simulink model "HFI_UB_counter_latch"  (R2024a)
settings: Solver=FixedStepAuto  StartTime=0.0  StopTime=10  FixedStep=1e-6  RelTol=1e-3
values from neighbouring files (symbols this model uses):
  flux = 0.005753    [HFI_AVi.sldd]
  Ld = 0.00025    [HFI_AVi.sldd]
  Lq = 0.00056    [HFI_AVi.sldd]
  R = 0.6    [HFI_AVi.sldd]
undefined symbols (not defined in the file or in its folder): DiscIntNeverNeededParam, PI
libraries: simulink x3, slpidlib x3, powerlib_extras x2, spsDCVoltageSourceLib x1, spsGroundLib x1, spsPermanentMagnetSynchronousMachineLib x1, spsUniversalBridgeLib x1, sps_lib x1
(part 2 of 2)

== system HFI_UB_counter_latch/FOC_Model/currloop/求定子电流矢量角/Id ~=0/id1<=0 ==
  In1 : Inport
  Action Port : ActionPort  ActionPortLabel=if(u1 <= 0)
  Out1 : Outport
  wires:
  In1/1 -> Out1/1

== system HFI_UB_counter_latch/FOC_Model/currloop/求定子电流矢量角/Id ~=0/id1>0 ==
  In1 : Inport
  Action Port : ActionPort  ActionPortLabel=else
  Out1 : Outport
  wires:
  In1/1 -> Out1/1

== system HFI_UB_counter_latch/FOC_Model/currloop/求定子电流矢量角/Id ~=0/id<=0 ==
  In1 : Inport
  Action Port : ActionPort  ActionPortLabel=if(u1 <= 0)
  Out1 : Outport
  wires:
  In1/1 -> Out1/1

== system HFI_UB_counter_latch/FOC_Model/currloop/求定子电流矢量角/Id ~=0/id>0 ==
  In1 : Inport
  Action Port : ActionPort  ActionPortLabel=else
  Out1 : Outport
  wires:
  In1/1 -> Out1/1

== matlab function HFI_UB_counter_latch/FOC_Model/currloop/polo/Subsystem4/CounterLatch150ms ==
  data: u input; y output
function y = fcn(u)
%#codegen
% Capture u once at 150 ms (Ts = 100 us) and hold it.
persistent sample_count latched_value
if isempty(sample_count)
    sample_count = uint16(0);
    latched_value = single(0);
end
if sample_count == uint16(1500)
    latched_value = single(u);
end
if sample_count < uint16(1501)
    sample_count = sample_count + uint16(1);
end
y = latched_value;
end

== matlab function HFI_UB_counter_latch/FOC_Model/currloop/SVPWM MATLAB Function ==
  data: Valpha input single size=1; Tcmp1 output single size=1; Vbeta input single size=1; Tcmp2 output single size=1; Tcmp3 output single size=1; Udc input single size=1; Tpwm input single size=1; sector output single size=1
function [Tcmp1,Tcmp2,Tcmp3,sector] = fcn(Valpha,Vbeta,Udc,Tpwm)
%#codegen

sector = single(0);
Tcmp1 = single(0);
Tcmp2 = single(0);
Tcmp3 = single(0);

%========Parameters statement================

    Vref1 = Vbeta;							                   
    Vref2 = (sqrt(3)*Valpha - Vbeta)/2; 				    
    Vref3 = (-sqrt(3)*Valpha - Vbeta)/2;					
   
 %========Sector calculation=================

  if (Vref1>0)
	   sector = single(1);
  end
  if (Vref2>0)
	   sector = sector+single(2);
  end
  if (Vref3>0)
       sector = sector+single(4);
  end

%======== X Y Z calculation===================

X = sqrt(3)*Vbeta*Tpwm/Udc;
Y = Tpwm/Udc*(3/2*Valpha+sqrt(3)/2*Vbeta);
Z = Tpwm/Udc*(-3/2*Valpha+sqrt(3)/2*Vbeta);	         

%==========Duty ratio calculation================
switch (sector)   
    case 1
        T1 = Z; T2 = Y; 
	case 2
        T1 = Y; T2 = -X; 
	case 3
        T1 = -Z; T2 = X; 
	case 4
        T1 = -X; T2 = Z;
	case 5
        T1 = X; T2 = -Y;
    otherwise
        T1 = -Y; T2 = -Z;
end

if T1+T2 > Tpwm
    T1 = T1/(T1+T2);
    T2 = T2/(T1+T2);
else
    T1 = T1;
    T2 = T2;
end
ta = (Tpwm-(T1+T2))/4.0;
tb = ta+T1/2;
tc = tb+T2/2;

%==========Duty ratio calculation================
switch (sector)
    case 1 
        Tcmp1=tb;
        Tcmp2=ta;
        Tcmp3=tc; 
        
    case 2 
        Tcmp1=ta;
        Tcmp2=tc;
        Tcmp3=tb; 
       
    case 3 
        Tcmp1=ta;
        Tcmp2=tb;
        Tcmp3=tc; 
        
    case 4 
        Tcmp1=tc;
        Tcmp2=tb;
        Tcmp3=ta;
        
    case 5 
        Tcmp1=tc;
        Tcmp2=ta;
        Tcmp3=tb;
        
   case 6
       Tcmp1=tb;
       Tcmp2=tc;
       Tcmp3=ta;
end
end

== matlab function HFI_UB_counter_latch/FOC_Model/currloop/MATLAB Function ==
  data: model_n input single size=1; hf_n input single size=1; n output single size=1; model_thetae input; hfi_thetae input; t input; thetae output; flag output; hfi_ready output; mode_out output
function [n, thetae, flag, hfi_ready, mode_out] = fcn( ...
    model_n, hf_n, model_thetae, hfi_thetae, t)
%#codegen

%% ================= 参数 =================
TS = single(1e-4);             % 100 us，10 kHz

HFI_BLEND_START = single(300); % 开始HFI-SMO融合
SMO_ENTER       = single(700); % 700 r/min以上才进入纯SMO
SMO_EXIT        = single(550); % 550 r/min以下退出纯SMO

ANGLE_MAX = single(pi/6);      % 最大角度差30°
SPEED_MAX = single(150);       % 最大速度差150 r/min

ENTER_CONFIRM = uint16(100);   % 10 ms
EXIT_CONFIRM  = uint16(100);   % 10 ms
VALID_CONFIRM = uint16(50);    % 5 ms
WAKE_SAMPLES  = uint16(200);   % 20 ms

T_BLEND     = single(0.05);    % 50 ms融合时间
LAMBDA_STEP = TS/T_BLEND;

PI     = single(pi);
TWO_PI = single(2*pi);

% mode:
% 0 = 纯HFI
% 1 = HFI向SMO融合
% 2 = 纯SMO
% 3 = HFI预唤醒，输出仍使用SMO
% 4 = SMO向HFI融合

%% ================= 状态变量 =================
persistent mode
persistent lambda_mem
persistent theta_prev
persistent enter_count
persistent exit_count
persistent valid_count
persistent wake_count

if isempty(mode)
    mode = uint8(0);
end

if isempty(lambda_mem)
    lambda_mem = single(0);
end

if isempty(theta_prev)
    theta_prev = single(0);
end

if isempty(enter_count)
    enter_count = uint16(0);
end

if isempty(exit_count)
    exit_count = uint16(0);
end

if isempty(valid_count)
    valid_count = uint16(0);
end

if isempty(wake_count)
    wake_count = uint16(0);
end

%% ============ HFI与SMO一致性检查 ============

% 最短角度差，范围为-pi～pi
dtheta = model_thetae - hfi_thetae;
dtheta = mod(dtheta + PI, TWO_PI) - PI;

angle_valid = abs(dtheta) < ANGLE_MAX;
speed_valid = abs(model_n - hf_n) < SPEED_MAX;

estimate_valid = angle_valid && speed_valid;

%% ================= 默认输出 =================
flag      = single(0);
hfi_ready = single(0);

%% ================= 启动阶段 =================
if t < single(0.3)

    mode       = uint8(0);
    lambda_mem = single(0);

    enter_count = uint16(0);
    exit_count  = uint16(0);
    valid_count = uint16(0);
    wake_count  = uint16(0);

    flag      = single(0);  % 完整HFI注入
    hfi_ready = single(1);

    theta_prev = hfi_thetae;

else

    switch mode

        %% ================ 纯HFI ================
        case 0

            lambda_mem = single(0);
            flag       = single(0);
            hfi_ready  = single(1);

            % 达到融合速度，而且两种观测器一致
            if abs(hf_n) >= HFI_BLEND_START && estimate_valid

                if enter_count < ENTER_CONFIRM
                    enter_count = enter_count + uint16(1);
                end

            else
                enter_count = uint16(0);
            end

            % 连续满足10 ms后进入融合
            if enter_count >= ENTER_CONFIRM

                mode = uint8(1);

                enter_count = uint16(0);
                valid_count = uint16(0);
            end

        %% ============ HFI向SMO融合 =============
        case 1

            hfi_ready = single(1);

            % 根据HFI速度计算目标融合权重
            x = (abs(hf_n) - HFI_BLEND_START)/ ...
                (SMO_ENTER - HFI_BLEND_START);

            x = min(max(x, single(0)), single(1));

            % 余弦平滑权重
            lambda_target = single(0.5) - ...
                single(0.5)*cos(PI*x);

            % 两种估算一致时才允许向目标权重变化
            if estimate_valid

                if lambda_mem < lambda_target

                    lambda_mem = min( ...
                        lambda_mem + LAMBDA_STEP, ...
                        lambda_target);

                elseif lambda_mem > lambda_target

                    lambda_mem = max( ...
                        lambda_mem - LAMBDA_STEP, ...
                        lambda_target);
                end

            else
                % 不一致时退回HFI
                lambda_mem = max( ...
                    lambda_mem - LAMBDA_STEP, ...
                    single(0));
            end

            % 解耦HFI注入幅值和角度融合权重：
            % lambda小于0.5时保持完整HFI注入；
            % lambda从0.5到1时再逐渐关闭HFI。
            if lambda_mem <= single(0.5)

                flag = single(0);

            else

                inject_x = ...
                    (lambda_mem-single(0.5))/single(0.5);

                inject_x = min(max( ...
                    inject_x, single(0)), single(1));

                flag = single(0.5) - ...
                    single(0.5)*cos(PI*inject_x);
            end

            % 满足条件后进入纯SMO
            if lambda_mem >= single(0.999) && ...
               abs(model_n) >= SMO_ENTER && ...
               estimate_valid

                if valid_count < VALID_CONFIRM
                    valid_count = valid_count + uint16(1);
                end

            else
                valid_count = uint16(0);
            end

            if valid_count >= VALID_CONFIRM

                mode       = uint8(2);
                lambda_mem = single(1);

                valid_count = uint16(0);
                exit_count  = uint16(0);

                flag      = single(1);
                hfi_ready = single(0);
            end

            % 速度重新降低时退回纯HFI
            if abs(hf_n) < HFI_BLEND_START && ...
               lambda_mem <= single(0.001)

                mode       = uint8(0);
                lambda_mem = single(0);

                enter_count = uint16(0);
                valid_count = uint16(0);
            end

        %% ================= 纯SMO ================
        case 2

            lambda_mem = single(1);
            flag       = single(1); % HFI关闭
            hfi_ready  = single(0);

            % 低于退出阈值持续10 ms
            if abs(model_n) < SMO_EXIT

                if exit_count < EXIT_CONFIRM
                    exit_count = exit_count + uint16(1);
                end

            else
                exit_count = uint16(0);
            end

            if exit_count >= EXIT_CONFIRM

                mode = uint8(3);

                exit_count  = uint16(0);
                wake_count  = uint16(0);
                valid_count = uint16(0);
                enter_count = uint16(0);
            end

        %% =============== HFI预唤醒 ===============
        case 3

            % 仍完全采用SMO角度
            lambda_mem = single(1);
            hfi_ready  = single(0);

            if wake_count < WAKE_SAMPLES
                wake_count = wake_count + uint16(1);
            end

            wake_x = single(wake_count)/ ...
                single(WAKE_SAMPLES);

            wake_x = min(max( ...
                wake_x, single(0)), single(1));

            wake_weight = single(0.5) - ...
                single(0.5)*cos(PI*wake_x);

            % flag从1降到0，HFI注入逐渐恢复
            flag = single(1)-wake_weight;

            % 如果速度重新升高，取消返回HFI
            if abs(model_n) >= SMO_ENTER

                if enter_count < ENTER_CONFIRM
                    enter_count = enter_count + uint16(1);
                end

            else
                enter_count = uint16(0);
            end

            if enter_count >= ENTER_CONFIRM

                mode       = uint8(2);
                lambda_mem = single(1);

                flag       = single(1);
                hfi_ready  = single(0);

                enter_count = uint16(0);
                wake_count  = uint16(0);
                valid_count = uint16(0);

            elseif wake_count >= WAKE_SAMPLES

                % HFI已经恢复，等待估算结果连续一致
                flag = single(0);

                if estimate_valid

                    if valid_count < VALID_CONFIRM
                        valid_count = valid_count + uint16(1);
                    end

                else
                    valid_count = uint16(0);
                end

                if valid_count >= VALID_CONFIRM

                    mode       = uint8(4);
                    lambda_mem = single(1);
                    hfi_ready  = single(1);

                    valid_count = uint16(0);
                end
            end

        %% ============ SMO向HFI融合 =============
        case 4

            flag      = single(0); % 保持完整HFI注入
            hfi_ready = single(1);

            if estimate_valid

                % 两种估算一致时才向HFI平滑切换
                lambda_mem = max( ...
                    lambda_mem-LAMBDA_STEP, ...
                    single(0));

            else
                % HFI失去可信度时停止切换，
                % 返回预唤醒/一致性确认状态
                mode       = uint8(3);
                lambda_mem = single(1);

                wake_count  = WAKE_SAMPLES;
                valid_count = uint16(0);

                flag      = single(0);
                hfi_ready = single(0);
            end

            if lambda_mem <= single(0.001)

                mode       = uint8(0);
                lambda_mem = single(0);

                enter_count = uint16(0);
                valid_count = uint16(0);
            end

        otherwise

            mode       = uint8(0);
            lambda_mem = single(0);

            enter_count = uint16(0);
            exit_count  = uint16(0);
            valid_count = uint16(0);
            wake_count  = uint16(0);

            flag      = single(0);
            hfi_ready = single(1);
    end
end

%% ================= 速度融合 =================
n = (single(1)-lambda_mem)*hf_n + ...
    lambda_mem*model_n;

%% ================= 角度融合 =================

% dtheta是HFI到SMO的最短角度差
theta_candidate = hfi_thetae + ...
    lambda_mem*dtheta;

%% ============== 保证输出角度连续 ==============

candidate_wrapped = mod(theta_candidate, TWO_PI);
previous_wrapped  = mod(theta_prev, TWO_PI);

theta_step = candidate_wrapped - previous_wrapped;
theta_step = mod(theta_step + PI, TWO_PI) - PI;

theta_continuous = theta_prev + theta_step;
theta_prev       = theta_continuous;

% Park变换继续使用0～2pi范围内的电角度
thetae = mod(theta_continuous, TWO_PI);

%% ================= 调试输出 =================
mode_out = single(mode);

end

== matlab function HFI_UB_counter_latch/FOC_Model/currloop/DirectionLatch ==
  data: hf_n input; direction output; hfi_ready input
function direction = fcn(hf_n, hfi_ready)
%#codegen

persistent dir_mem
persistent positive_count
persistent negative_count

if isempty(dir_mem)
    dir_mem = single(1);
end

if isempty(positive_count)
    positive_count = uint16(0);
end

if isempty(negative_count)
    negative_count = uint16(0);
end

SPEED_THRESHOLD = single(50);
CONFIRM_COUNT = uint16(50); % 5 ms，模块按10 kHz执行

if hfi_ready > single(0.5)

    if hf_n > SPEED_THRESHOLD

        negative_count = uint16(0);

        if positive_count < CONFIRM_COUNT
            positive_count = positive_count + uint16(1);
        end

        if positive_count >= CONFIRM_COUNT
            dir_mem = single(1);
        end

    elseif hf_n < -SPEED_THRESHOLD

        positive_count = uint16(0);

        if negative_count < CONFIRM_COUNT
            negative_count = negative_count + uint16(1);
        end

        if negative_count >= CONFIRM_COUNT
            dir_mem = single(-1);
        end

    else
        positive_count = uint16(0);
        negative_count = uint16(0);
    end

else
    positive_count = uint16(0);
    negative_count = uint16(0);
end

direction = dir_mem;

end

== matlab function HFI_UB_counter_latch/MATLAB Function ==
  data: carrier input; g output; Tcm1 input; Tcm2 input; Tcm3 input; db input
function g = fcn(carrier, Tcm1, Tcm2, Tcm3, db)
%#codegen
% 三相中心对齐PWM死区生成
%
% 输入：
%   carrier  三角载波，范围为0～Tpwm/2，单位：s
%   Tcm1     A相比较值，单位：s
%   Tcm2     B相比较值，单位：s
%   Tcm3     C相比较值，单位：s
%   db       实际死区时间，单位：s
%
% 输出：
%   g(1) = A相上管
%   g(2) = A相下管
%   g(3) = B相上管
%   g(4) = B相下管
%   g(5) = C相上管
%   g(6) = C相下管
%
% 原理：
%   carrier >= Tcm + db/2：上管导通
%   carrier <= Tcm - db/2：下管导通
%   中间宽度为db的区域：上下管全部关闭
%
% 因此输入db=1e-6时，实际死区为1 μs。

%% 初始化输出

g = zeros(6,1);

% 防止输入负的死区时间
if db < 0
    db = 0;
end

% 比较值两侧各移动半个死区时间
half_db = db / 2;

%% A相桥臂

if carrier >= (Tcm1 + half_db)

    % A相上管导通，下管关闭
    g(1) = 1;
    g(2) = 0;

elseif carrier <= (Tcm1 - half_db)

    % A相上管关闭，下管导通
    g(1) = 0;
    g(2) = 1;

else

    % 死区期间上下管全部关闭
    g(1) = 0;
    g(2) = 0;

end

%% B相桥臂

if carrier >= (Tcm2 + half_db)

    % B相上管导通，下管关闭
    g(3) = 1;
    g(4) = 0;

elseif carrier <= (Tcm2 - half_db)

    % B相上管关闭，下管导通
    g(3) = 0;
    g(4) = 1;

else

    % 死区期间上下管全部关闭
    g(3) = 0;
    g(4) = 0;

end

%% C相桥臂

if carrier >= (Tcm3 + half_db)

    % C相上管导通，下管关闭
    g(5) = 1;
    g(6) = 0;

elseif carrier <= (Tcm3 - half_db)

    % C相上管关闭，下管导通
    g(5) = 0;
    g(6) = 1;

else

    % 死区期间上下管全部关闭
    g(5) = 0;
    g(6) = 0;

end

end

== matlab function HFI_UB_counter_latch/MATLAB Function1 ==
  data: MtrPos input; actual_deg output; thetae input; est_deg output; error_deg output
function [actual_deg, est_deg, error_deg] = fcn(MtrPos, thetae)
%#codegen

Pn = single(4);
PI = single(pi);
TWO_PI = single(2*pi);

% 电机实际机械角度 → 实际电角度
theta_actual_e = mod(Pn*MtrPos, TWO_PI);

% 观测器电角度
theta_est_e = mod(thetae, TWO_PI);

% 计算最短电角度误差，范围为-pi～pi
error_rad = mod(theta_est_e-theta_actual_e+PI, TWO_PI)-PI;

% 转换成角度制，方便Scope观察
actual_deg = theta_actual_e*single(180/pi);
est_deg    = theta_est_e*single(180/pi);
error_deg  = error_rad*single(180/pi);

end
